simulink model "test_system_setup"  (R2025b)
settings: Solver=FixedStepDiscrete  StartTime=0.0  StopTime=inf  FixedStep=0.01  RelTol=1e-3
libraries: arduinolib x4, arduinosensorlib x1, mcbhdlcontrolslib x1, mcbhdlpositiondecoderlib x1, motor_control_lib x1
settings Model: ExtModeTrigDuration=2  Creator=ali89  LastModifiedBy=ali89
settings SolverCC: AutoInsertRateTranBlk=on
settings OptimizationCC: EnhancedBackFolding=on  PassReuseOutputArgsAs=Individual arguments  ZeroExternalMemoryAtStartup=off  ZeroInternalMemoryAtStartup=off  MaxStackSize=64  OptimizeBlockOrder=speed  DifferentSizesBufferReuse=on  OptimizationCustomize=off  EfficientTunableParamExpr=on
settings DebuggingCC: ParameterTunabilityLossMsg=error
settings HardwareCC: ProdBitPerPointer=32.0  ProdBitPerSizeT=32.0  ProdBitPerPtrDiffT=32.0  ProdLargestAtomicInteger=Long  ProdLargestAtomicFloat=Double  ProdWordSize=32.0  ProdHWDeviceType=ARM Compatible->ARM Cortex
settings SFSimCC: MATLABDynamicMemAlloc=off
settings RTWCC: SystemTargetFile=ert.tlc  HardwareBoard=ESP32-WROOM (Arduino Compatible)  TLCOptions="-aInlineSetEventsForThisBaseRateFcn=TLC_FALSE -aSuppressMultiTaskScheduler=TLC_FALSE  -aRateBasedStepFcn=0"  TemplateMakefile=ert_default_tmf  Toolchain=ESP32  Description=Embedded Coder
settings CodeAppCC: ForceParamTrailComments=on  IgnoreCustomStorageClasses=off  OperatorAnnotations=on  SimulinkDataObjDesc=on  SFDataObjDesc=on  InsertBlockDesc=on
settings ERTTargetCC: ExtModeTransport=3.0  ExtModeStaticAlloc=on  ExtModeAutomaticAllocSize=off  ExtModeStaticAllocSize=65536.0  ExtModeMexFile=ext_xcp  ExtModeIntrfLevel=Level2 - Open  InlinedParameterPlacement=Hierarchical  SupportContinuousTime=on  SupportVariableSizeSignals=on

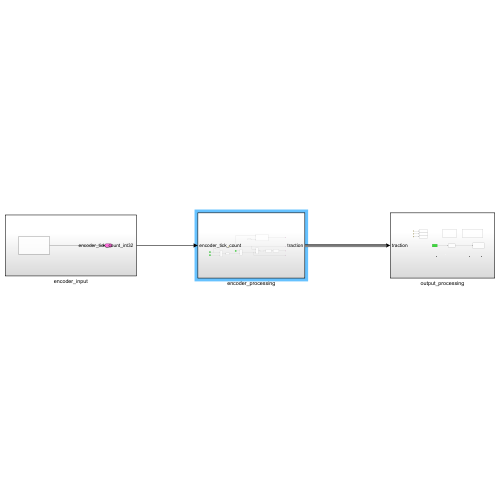
[thumbnail: Simulink's stored preview of the top-level diagram]
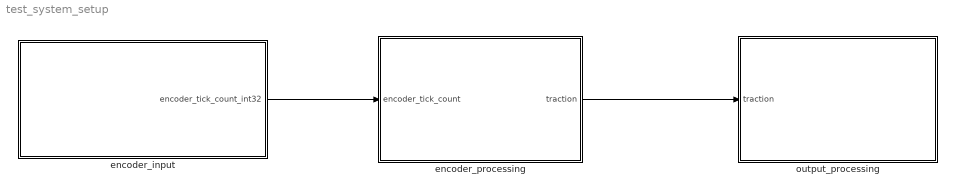
== system test_system_setup ==
  encoder_input : Subsystem
  encoder_processing : Subsystem
  output_processing : Subsystem
  wires:
  encoder_input/1("encoder_tick_count_int32 ") -> encoder_processing/1(encoder_tick_count)
  encoder_processing/1(traction) -> output_processing/1(traction)

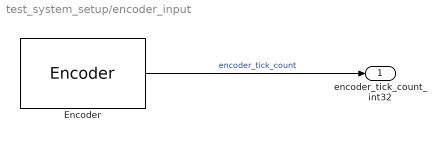
== system test_system_setup/encoder_input ==
  Encoder : arduinosensorlib/Encoder  InputA=25  InputB=26  Mode=No reset  SampleTime=-1
  "encoder_tick_count_int32 " : Outport
  wires:
  Encoder/1 -> "encoder_tick_count_int32 "/1  "encoder_tick_count"

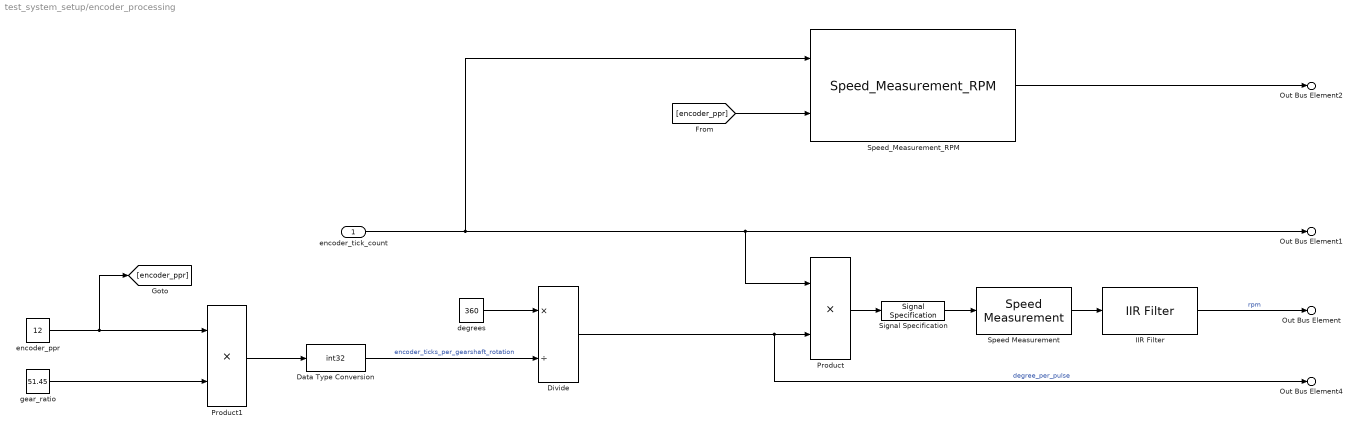
== system test_system_setup/encoder_processing ==
  encoder_tick_count : Inport
  Data Type Conversion : DataTypeConversion  OutDataTypeStr=int32  SaturateOnIntegerOverflow=off  RndMeth=Floor
  Divide : Product  Inputs=*/
  IIR Filter : mcbhdlcontrolslib/IIR Filter  VariantControl=Low Pass Filter  VariantSelect=Low-pass  FilterConstantInputType=Specify via dialog  Filter_constant=0.01  advancedSettings=off  Ts=50e-6  cutOff_freq=32.1525
      settings: LibrarySourceBlock=mcbhdllib/Signal Management/IIR Filter
  Product : Product
  Product1 : Product
  Signal Specification : SignalSpecification  Unit=deg
  Speed Measurement : mcbhdlpositiondecoderlib/Speed Measurement  PositionUnit=Degrees  PositionScalingDatatype=uint32  SpeedCalculationMode=Maximum application speed  SampleTimeAsync=0.01  MaximumApplicationSpeed=33000  SpeedResolution=5e-6  DelayLength=1  MaximumMeasurableSpeed=1500  MeasurableSpeedResolution=6.9849e-07  SpeedUnit=RPM  PerUnitSpeed=1000  SpeedDataType=single
      settings: LibrarySourceBlock=mcbhdllib/Sensor Decoders/Speed Measurement
  Speed_Measurement_RPM : motor_control_lib/Speed_Measurement_RPM  SystemSampleTime=-1  VariantActivationTime=update diagram  EmptyChoice=off  PassThrough=off  PassThroughVariantControl=(default)  EmptyChoiceVariantControl=(default)  AllowFlexibleInterface=on  Latency=0  AutoFrameSizeCalculation=off
  degrees : Constant  Value=360
  encoder_ppr : Constant  Value=12
  gear_ratio : Constant  Value=51.45
  Out Bus Element : Outport  PortName=traction  Element=gear_shaft_rpm
  Out Bus Element1 : Outport  PortName=traction  Element=encoder_tick_count
  Out Bus Element2 : Outport  PortName=traction  Element=motor_shaft_rpm
  Out Bus Element4 : Outport  PortName=traction  Element=gear_shaft_degree_per_pulse
  wires:
  Divide/1 -> Out Bus Element4/1, Product/2  "degree_per_pulse"
  Product/1 -> Signal Specification/1
  Signal Specification/1 -> Speed Measurement/1
  Speed Measurement/1 -> IIR Filter/1
  IIR Filter/1 -> Out Bus Element/1  "rpm"
  encoder_ppr/1 -> [encoder_ppr], Product1/1
  gear_ratio/1 -> Product1/2
  degrees/1 -> Divide/1
  Product1/1 -> Data Type Conversion/1
  Data Type Conversion/1 -> Divide/2  "encoder_ticks_per_gearshaft_rotation"
  encoder_tick_count/1 -> Speed_Measurement_RPM/1, Out Bus Element1/1, Product/1
  [encoder_ppr] -> Speed_Measurement_RPM/2
  Speed_Measurement_RPM/1 -> Out Bus Element2/1

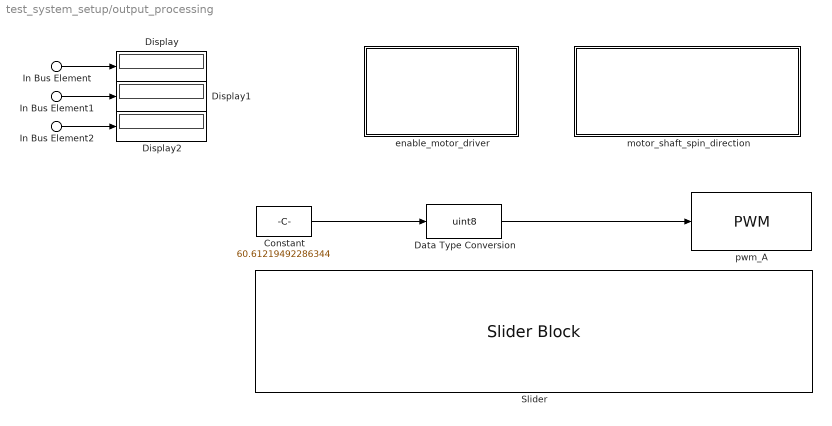
== system test_system_setup/output_processing ==
  In Bus Element : Inport  PortName=traction  Element=encoder_tick_count
  In Bus Element1 : Inport  PortName=traction  Element=gear_shaft_rpm
  In Bus Element2 : Inport  PortName=traction  Element=motor_shaft_rpm
  Constant : Constant  Value=60.61219492286344
  Data Type Conversion : DataTypeConversion  OutDataTypeStr=uint8  SaturateOnIntegerOverflow=off  RndMeth=Floor
  Display : Display
  Display1 : Display
  Display2 : Display
  Slider : SliderBlock  LabelPosition=Hide  ScaleMax=255
  enable_motor_driver : Subsystem
  motor_shaft_spin_direction : Subsystem
  pwm_A : arduinolib/PWM  pinNumber=23  frequencyType=Specify  desiredFrequency=150  achievableFrequency=150
  wires:
  Data Type Conversion/1 -> pwm_A/1
  Constant/1 -> Data Type Conversion/1
  In Bus Element/1 -> Display/1
  In Bus Element1/1 -> Display1/1
  In Bus Element2/1 -> Display2/1

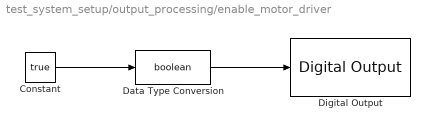
== system test_system_setup/output_processing/enable_motor_driver ==
  Constant : Constant  Value=true
  Data Type Conversion : DataTypeConversion  OutDataTypeStr=boolean  SaturateOnIntegerOverflow=off  RndMeth=Floor
  Digital Output : arduinolib/Digital Output  pinNumber=4  Direction=output  blockPlatform=arduino
  wires:
  Constant/1 -> Data Type Conversion/1
  Data Type Conversion/1 -> Digital Output/1

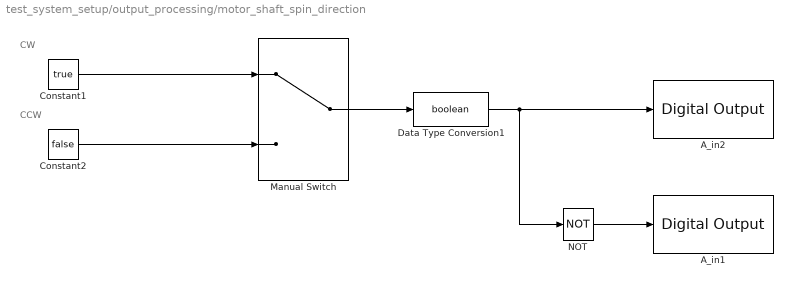
== system test_system_setup/output_processing/motor_shaft_spin_direction ==
  note: CCW
  note: CW
  A_in1 : arduinolib/Digital Output  pinNumber=17  Direction=output  blockPlatform=arduino
  A_in2 : arduinolib/Digital Output  pinNumber=22  Direction=output  blockPlatform=arduino
  Constant1 : Constant  Value=true
  Constant2 : Constant  Value=false
  Data Type Conversion1 : DataTypeConversion  OutDataTypeStr=boolean  SaturateOnIntegerOverflow=off  RndMeth=Floor
  Manual Switch : ManualSwitch
  NOT : Logic  Operator=NOT  AllPortsSameDT=off  OutDataTypeStr=boolean
  wires:
  Data Type Conversion1/1 -> NOT/1, A_in2/1
  NOT/1 -> A_in1/1
  Manual Switch/1 -> Data Type Conversion1/1
  Constant1/1 -> Manual Switch/1
  Constant2/1 -> Manual Switch/2
